simulink model "mark3"  (R2016a)
settings: Solver=VariableStepAuto  StartTime=0.0  StopTime=10  RelTol=1e-3
libraries: vrlib x2
settings Model: Creator=Prajesh Sanghvi  LastModifiedBy=Prajesh Sanghvi

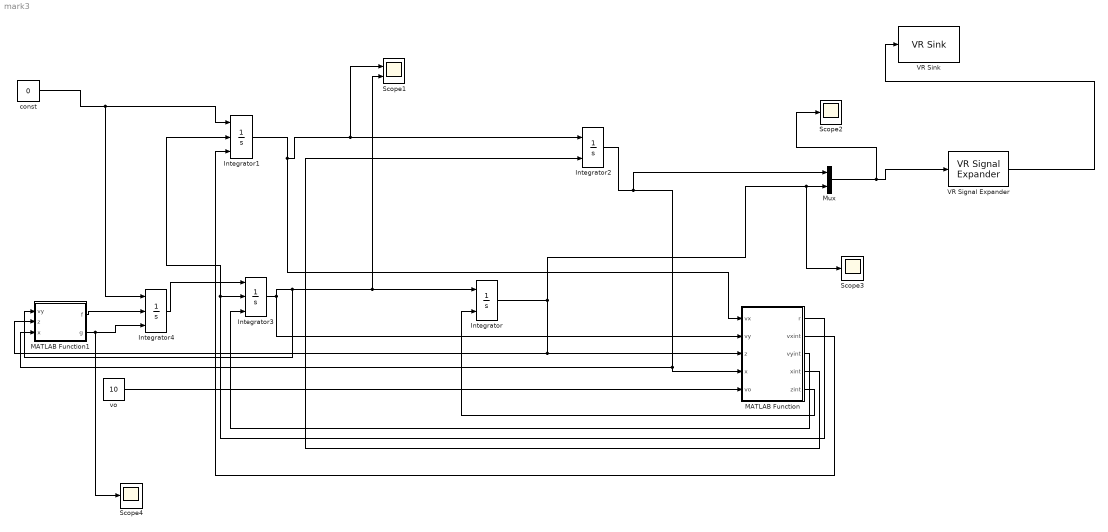
== system mark3 ==
  Integrator : Integrator  InitialConditionSource=external
  Integrator1 : Integrator  ExternalReset=rising  InitialConditionSource=external
  Integrator2 : Integrator  InitialConditionSource=external
  Integrator3 : Integrator  ExternalReset=rising  InitialConditionSource=external
  Integrator4 : Integrator  ExternalReset=rising  InitialConditionSource=external
  MATLAB Function : MATLAB Function  TreatAsAtomicUnit=on
  MATLAB Function1 : MATLAB Function  TreatAsAtomicUnit=on
  Mux : Mux  Inputs=2
  Scope1 : Scope  NumInputPorts=2
  Scope2 : Scope
  Scope3 : Scope
  Scope4 : Scope
  VR Signal Expander : vrlib/VR Signal Expander  outwidth=3  outidx=[3 2]
  VR Sink : vrlib/VR Sink  InstantiateOnLoad=on  SampleTime=0.001  ViewEnable=on  RemoteChange=off  RemoteView=off  FieldsWritten=disk.translation.3.1.1.double  WorldFileName=C:\Users\Prajesh Sanghvi\Desktop\folders\robocon\arina.wrl  AutoView=off  VideoDimensions=[]  AllowVariableSize=off
  const : Constant  Value=0
  vo : Constant  Value=10
  wires:
  MATLAB Function/2(vxint) -> Integrator1/3
  MATLAB Function/3(vyint) -> Integrator3/3
  MATLAB Function/4(xint) -> Integrator2/2
  MATLAB Function/5(zint) -> Integrator/2
  Integrator2/1 -> MATLAB Function1/3(x), MATLAB Function/4(x), Mux/1
  Integrator/1 -> Scope3/1, Mux/2, MATLAB Function/3(z), MATLAB Function1/2(z)
  Integrator1/1 -> MATLAB Function/1(vx), Scope1/1, Integrator2/1
  Integrator3/1 -> MATLAB Function1/1(vy), Scope1/2, Integrator/1, MATLAB Function/2(vy)
  const/1 -> Integrator4/1, Integrator1/1
  vo/1 -> MATLAB Function/5(vo)
  Mux/1 -> Scope2/1, VR Signal Expander/1
  MATLAB Function/1(r) -> Integrator1/2, Integrator3/2
  MATLAB Function1/1(f) -> Integrator4/2
  MATLAB Function1/2(g) -> Integrator4/3, Scope4/1
  Integrator4/1 -> Integrator3/1
  VR Signal Expander/1 -> VR Sink/1

== matlab function mark3/MATLAB Function1 ==
  data: f output; vy input; g output; z input; x input
function [f,g] = fcn(vy,z,x)
% vyf=vy;
g=-9.8;
f=1;
if(x>=3)
    g=0;
end
if(z<=1)
 %if(abs(vy)<=.0001)
     g=0;
     vy=0;
   %  vyf=vy; 
     f=-1;
 %end
end

== matlab function mark3/MATLAB Function ==
  data: r output; vx input; vxint output; vy input; z input; x input; vyint output; xint output; zint output; vo input
function [r,vxint,vyint,xint,zint] = fcn(vx,vy,z,x,vo)


    
vxint=vo*cos(pi/3);
vyint=vo*sin(pi/3);
xint=-6;
zint=0.9;

  r=1;
 %if z<=14.5 && z>=0
 if z>=0.9
    r=-1;
 end
 
 
 %if z==-6
   if x>=3
       
   % xint=0;
    %zint=0;
      vxint=0;
       vyint=0;
   % r=1;
    end
% end
